simulink subsystem "continuous_time_controller"  (R2020b)
settings: Solver=VariableStepAuto  StartTime=0.0  StopTime=10.0  RelTol=1e-3
model mask{lambda=0, forward_action_enabled=on}
values from neighbouring files (symbols this model uses):
  forward_action_enabled = false    [buildFunDV_lambda.m]    (also in opt_problem_lambda.m)
  lambda = fmincon(fun,lambda_0,[],[],[],[],0,lambda_MAX, [], options)    [opt_problem_lambda.m]
settings Model: Creator=marco  LastModifiedBy=marco

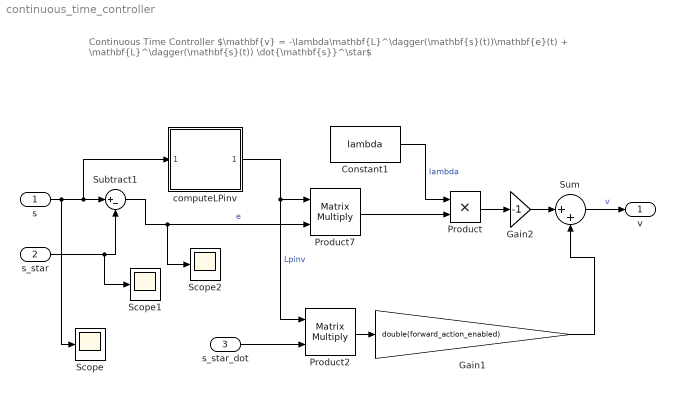
== system continuous_time_controller ==
  note: Continuous Time Controller
      | $\mathbf{v} = -\lambda\mathbf{L}^\dagger(\mathbf{s}(t))\mathbf{e}(t) + \mathbf{L}^\dagger(\mathbf{s}(t)) \dot{\mathbf{s}}^\star$
  s : Inport
  s_star : Inport  Port=2
  s_star_dot : Inport  Port=3
  Constant1 : Constant  Value=lambda
  Gain1 : Gain  Gain=double(forward_action_enabled)
  Gain2 : Gain  Gain=-1
  Product : Product
  Product2 : Product  Multiplication=Matrix(*)
  Product7 : Product  Multiplication=Matrix(*)
  Scope : Scope
  Scope1 : Scope
  Scope2 : Scope
  Subtract1 : Sum  Inputs=|+-
  Sum : Sum  Inputs=|++
  computeLPinv : Subsystem  ReferencedSubsystem=computeLPinv
  v : Outport
  wires:
  computeLPinv/1 -> Product2/1, Product7/1  "Lpinv"
  Sum/1 -> v/1  "v"
  Product7/1 -> Product/2
  Gain2/1 -> Sum/1
  Product/1 -> Gain2/1
  Constant1/1 -> Product/1  "lambda"
  s/1 -> Subtract1/1, computeLPinv/1, Scope/1
  s_star/1 -> Subtract1/2, Scope1/1
  Subtract1/1 -> Product7/2, Scope2/1  "e"
  s_star_dot/1 -> Product2/2
  Product2/1 -> Gain1/1
  Gain1/1 -> Sum/2
